simulink model "work2"  (R2020b)
settings: Solver=ode15s  StartTime=0.0  StopTime=50  MaxStep=le-2  RelTol=1e-3
settings Model: Creator=75252  LastModifiedBy=zhiyao
settings DebuggingCC: UnconnectedInputMsg=none  UnconnectedOutputMsg=none  UnconnectedLineMsg=none
settings ModelReferenceCC: EnableRefExpFcnMdlSchedulingChecks=off

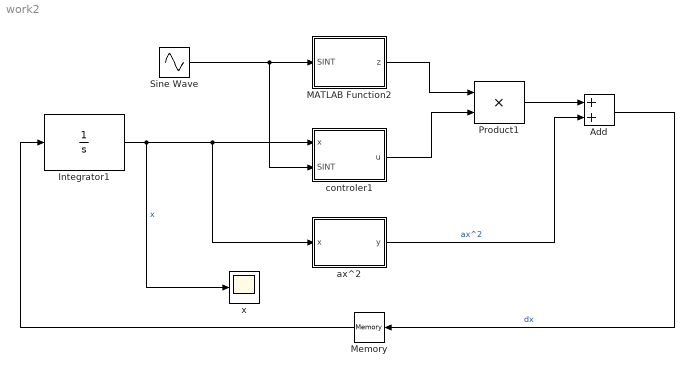
== system work2 ==
  Add : Sum
  Integrator1 : Integrator  InitialCondition=1
  MATLAB Function2 : MATLAB Function  TreatAsAtomicUnit=on
  Memory : Memory
  Product1 : Product
  Sine Wave : Sin  SampleTime=0
  ax^2 : MATLAB Function  TreatAsAtomicUnit=on
  controler1 : MATLAB Function  TreatAsAtomicUnit=on
  x : Scope
  wires:
  MATLAB Function2/1(z) -> Product1/1
  controler1/1(u) -> Product1/2
  Integrator1/1 -> x/1, ax^2/1(x), controler1/1(x)  "x"
  Product1/1 -> Add/1
  ax^2/1(y) -> Add/2  "ax^2"
  Add/1 -> Memory/1  "dx"
  Sine Wave/1 -> controler1/2(SINT), MATLAB Function2/1(SINT)
  Memory/1 -> Integrator1/1

== matlab function work2/controler1 ==
  data: x input; u output; SINT input
function u = fcn(x,SINT)
a=1;b=1;c=1;k=1;

u = (-k*x-a*x^2)*(b+c*SINT^2);

== matlab function work2/ax^2 ==
  data: x input; y output
function y = fcn(x)
a=1;
y = a*x^2;

== matlab function work2/MATLAB Function2 ==
  data: z output; SINT input
function z = fcn(SINT)
b=1;c=1;
z = 1/(b+c*SINT);
